simulink model "motorcontrol_19a"  (R2019a)
settings: Solver=FixedStepDiscrete  StartTime=0.0  StopTime=20  FixedStep=Ts.simulink  MaxStep=5e-5  RelTol=1e-3  EnableMultiTasking=on
undefined symbols (not defined in the file): ControllerMode, ControlMode, ctrlParams, dataType, DiscIntNeverNeededParam, inverter, NumBits1, NumBits2, PI_params, pmsm, Slope1, Slope2, Ts
libraries: simulink x17
(part 2 of 3)

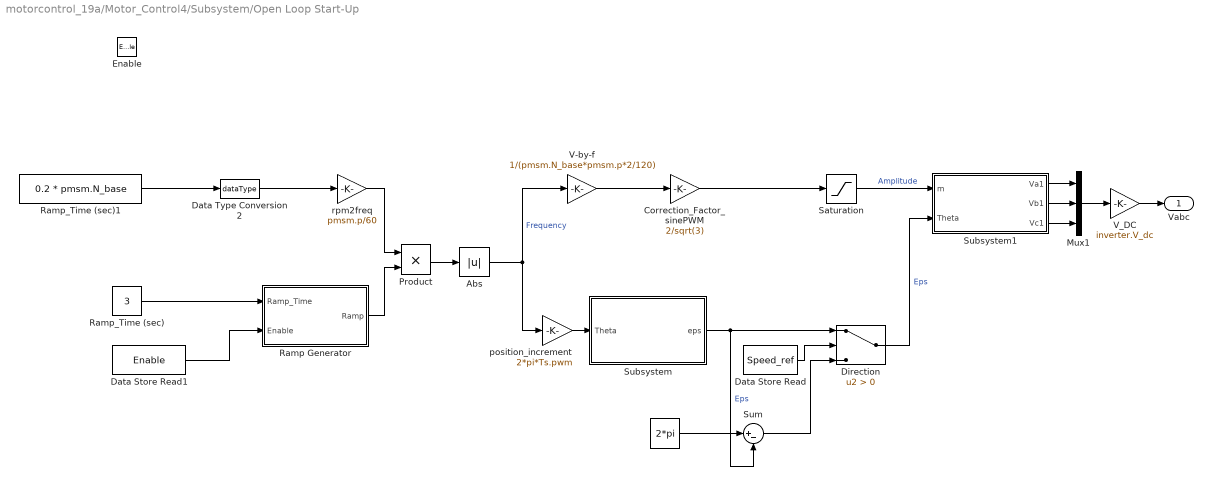
== system motorcontrol_19a/Motor_Control4/Subsystem/Open Loop Start-Up ==
  Enable : EnablePort  StatesWhenEnabling=reset
  " " : Constant  Value=2*pi  OutDataTypeStr=dataType  SampleTime=-1
  Abs : Abs
  Correction_Factor_sinePWM : Gain  Gain=2/sqrt(3)  RndMeth=Simplest  OutDataTypeStr=Inherit: Same as input
  Data Store Read : DataStoreRead  DataStoreName=Speed_ref
  Data Store Read1 : DataStoreRead  DataStoreName=Enable
  Data Type Conversion2 : DataTypeConversion  OutDataTypeStr=dataType  RndMeth=Simplest
  Direction : Switch  Criteria=u2 > Threshold  OutDataTypeStr=dataType  RndMeth=Simplest
  Mux1 : Mux  Inputs=3
  Product : Product  RndMeth=Simplest  OutDataTypeStr=Inherit: Same as first input
  Ramp Generator : Subsystem
  Ramp_Time (sec) : Constant  Value=3  OutDataTypeStr=dataType  SampleTime=-1
  Ramp_Time (sec)1 : Constant  Value=0.2 * pmsm.N_base  OutDataTypeStr=dataType  SampleTime=-1
  Saturation : Saturate  UpperLimit=0.95  LowerLimit=0.15  RndMeth=Simplest
  Subsystem : Subsystem  mask(Position Generator){Offset=0, InitialCondition=0}
      mask prompts: Offset "Initial Theta output:"; InitialCondition "Initial condition"
      mask help:
      | <p>Generate position ramp of required frequency.
      | <br><br>
      | The block accepts position increment and outputs position ramp.
      | <br>
      | The position increment for required frequency (Hz) can be computed by following:
      | <br><br>
      | &Delta;&theta; (per-unit) = Frequency&#8231;Sample Time
      | <br>
      | &Delta;&theta; (radians)&nbsp; = 2&#8231;&pi;&#8231;Frequency&#8231;Sample Time
      | <br>
      | &Delta;&theta; (degrees) = 360&#8231;Frequency&#8231;Sample Time <br>
      mask Display: fprintf('Position\n Generator');
  Subsystem1 : Subsystem  mask(3-Phase Sine Voltage Generator){}
      mask help:
      | Generate balanced 3-phase sinusoidal signals described by magnitude and position inputs.
      |
      | The block accepts voltage reference by magnitude and position inputs, and outputs balanced three phase sinusoidal voltages of frequency corresponding to position input.
      |
      | Enter position input units and number of data points for sine-cosine look-up table.
      mask Display: fprintf('3-Phase Sine\n  Voltage Generator');
  Sum : Sum  Inputs=|+-  RndMeth=Simplest  OutDataTypeStr=Inherit: Same as first input
  V-by-f : Gain  Gain=1/(pmsm.N_base*pmsm.p*2/120)  RndMeth=Simplest  OutDataTypeStr=Inherit: Same as input
  V_DC : Gain  Gain=inverter.V_dc
  position_increment : Gain  Gain=2*pi*Ts.pwm  RndMeth=Simplest  OutDataTypeStr=Inherit: Same as input
  rpm2freq : Gain  Gain=pmsm.p/60  RndMeth=Simplest  OutDataTypeStr=Inherit: Same as input
  Vabc : Outport  VectorParamsAs1DForOutWhenUnconnected=off
  wires:
  V_DC/1 -> Vabc/1
  Data Store Read/1 -> Direction/2
  Ramp_Time (sec)1/1 -> Data Type Conversion2/1
  Data Type Conversion2/1 -> rpm2freq/1
  Correction_Factor_sinePWM/1 -> Saturation/1
  Data Store Read1/1 -> Ramp Generator/2(Enable)
  rpm2freq/1 -> Product/1
  Product/1 -> Abs/1
  V-by-f/1 -> Correction_Factor_sinePWM/1
  position_increment/1 -> Subsystem/1(Theta)
  Abs/1 -> V-by-f/1, position_increment/1  "Frequency"
  Sum/1 -> Direction/3
  " "/1 -> Sum/1
  Subsystem/1(eps) -> Direction/1, Sum/2  "Eps"
  Ramp_Time (sec)/1 -> Ramp Generator/1(Ramp_Time)
  Ramp Generator/1(Ramp) -> Product/2
  Mux1/1 -> V_DC/1
  Saturation/1 -> Subsystem1/1(m)  "Amplitude"
  Direction/1 -> Subsystem1/2(Theta)  "Eps"
  Subsystem1/2(Vb1) -> Mux1/2
  Subsystem1/1(Va1) -> Mux1/1
  Subsystem1/3(Vc1) -> Mux1/3

== system motorcontrol_19a/Subsystem/Simulation/Data_Type_Float ==
  In1 : Inport
  In2 : Inport  Port=2
  Data Type Conversion2 : DataTypeConversion  OutDataTypeStr=dataType  RndMeth=Simplest
  Mux : Mux  Inputs=2
  Data : Outport
  wires:
  Data Type Conversion2/1 -> Mux/2
  In2/1 -> Data Type Conversion2/1
  Mux/1 -> Data/1
  In1/1 -> Mux/1

== system motorcontrol_19a/Subsystem/Simulation/Parse ==
  Enable_PWM : Inport
  Bitwise Operator : simulink/Logic and Bit Operations/Bitwise Operator  logicop=AND  UseBitMask=on  BitMask=hex2dec('0001')  BitMaskRealWorld=Stored Integer
  Data : Outport
  wires:
  Enable_PWM/1 -> Bitwise Operator/1
  Bitwise Operator/1 -> Data/1

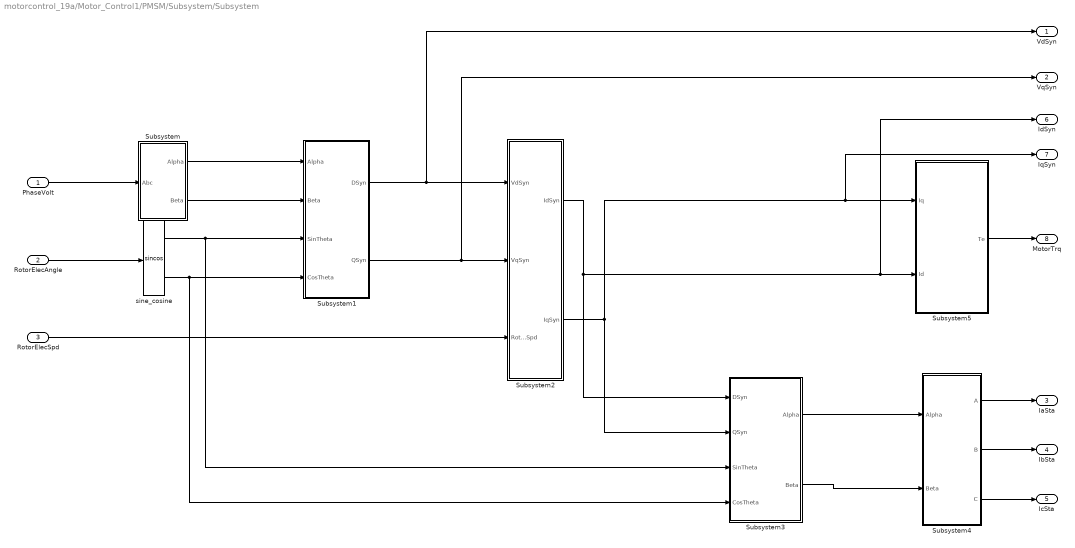
== system motorcontrol_19a/Motor_Control1/PMSM/Subsystem/Subsystem ==
  PhaseVolt : Inport
  RotorElecAngle : Inport  Port=2
  RotorElecSpd : Inport  Port=3
  Subsystem : Subsystem
  Subsystem1 : Subsystem
  Subsystem2 : Subsystem
  Subsystem3 : Subsystem
  Subsystem4 : Subsystem
  Subsystem5 : Subsystem
  sine_cosine : Trigonometry  Operator=sincos
  VdSyn : Outport  VectorParamsAs1DForOutWhenUnconnected=off
  VqSyn : Outport  Port=2  VectorParamsAs1DForOutWhenUnconnected=off
  IaSta : Outport  Port=3  VectorParamsAs1DForOutWhenUnconnected=off
  IbSta : Outport  Port=4  VectorParamsAs1DForOutWhenUnconnected=off
  IcSta : Outport  Port=5  VectorParamsAs1DForOutWhenUnconnected=off
  IdSyn : Outport  Port=6  VectorParamsAs1DForOutWhenUnconnected=off
  IqSyn : Outport  Port=7  VectorParamsAs1DForOutWhenUnconnected=off
  MotorTrq : Outport  Port=8  VectorParamsAs1DForOutWhenUnconnected=off
  wires:
  Subsystem4/2(B) -> IbSta/1
  Subsystem5/1(Te) -> MotorTrq/1
  Subsystem3/1(Alpha) -> Subsystem4/1(Alpha)
  Subsystem4/3(C) -> IcSta/1
  sine_cosine/1 -> Subsystem3/3(SinTheta), Subsystem1/3(SinTheta)
  Subsystem1/2(QSyn) -> VqSyn/1, Subsystem2/2(VqSyn)
  Subsystem3/2(Beta) -> Subsystem4/2(Beta)
  Subsystem2/2(IqSyn) -> IqSyn/1, Subsystem5/1(Iq), Subsystem3/2(QSyn)
  Subsystem4/1(A) -> IaSta/1
  RotorElecSpd/1 -> Subsystem2/3(RotorElecSpd)
  Subsystem/1(Alpha) -> Subsystem1/1(Alpha)
  Subsystem1/1(DSyn) -> Subsystem2/1(VdSyn), VdSyn/1
  Subsystem/2(Beta) -> Subsystem1/2(Beta)
  RotorElecAngle/1 -> sine_cosine/1
  sine_cosine/2 -> Subsystem3/4(CosTheta), Subsystem1/4(CosTheta)
  PhaseVolt/1 -> Subsystem/1(Abc)
  Subsystem2/1(IdSyn) -> Subsystem3/1(DSyn), IdSyn/1, Subsystem5/2(Id)

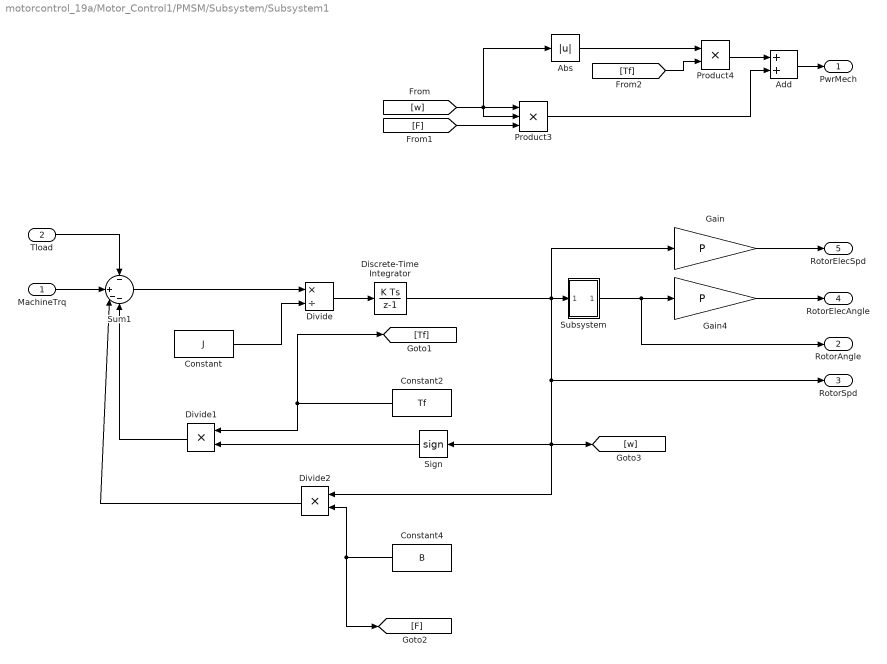
== system motorcontrol_19a/Motor_Control1/PMSM/Subsystem/Subsystem1 ==
  MachineTrq : Inport
  Tload : Inport  Port=2
  Abs : Abs
  Add : Sum
  Constant : Constant  Value=J  OutDataTypeStr=Inherit: Inherit via back propagation  SampleTime=-1
  Constant2 : Constant  Value=Tf  OutDataTypeStr=Inherit: Inherit via back propagation  SampleTime=-1
  Constant4 : Constant  Value=B  OutDataTypeStr=Inherit: Inherit via back propagation  SampleTime=-1
  Discrete-Time Integrator : DiscreteIntegrator  InitialCondition=omega_init  SampleTime=Ts  OutDataTypeStr=single  LimitOutput=on  UpperSaturationLimit=10e6  LowerSaturationLimit=-10e6  ICPrevOutput=DiscIntNeverNeededParam  ICPrevScaledInput=DiscIntNeverNeededParam
  Divide : Product  Inputs=*/  OutDataTypeStr=Inherit: Same as first input
  Divide1 : Product  Inputs=**
  Divide2 : Product  Inputs=**
  Gain : Gain  Gain=P  SaturateOnIntegerOverflow=on  OutDataTypeStr=Inherit: Same as input  ParamDataTypeStr=Inherit: Same as input
  Gain4 : Gain  Gain=P  SaturateOnIntegerOverflow=on  OutDataTypeStr=Inherit: Same as input  ParamDataTypeStr=Inherit: Same as input
  Product3 : Product  Inputs=3  OutDataTypeStr=Inherit: Inherit via back propagation
  Product4 : Product
  Sign : Signum
  Subsystem : Subsystem  mask{Ts=Ts, Ic=theta_init, U=pi, L=-pi}
      mask prompts: Ts "Sample Time:"; Ic "Initial Condition:"; U "Upper Limit:"; L "Lower Limit:"
  Sum1 : Sum  Inputs=-|+--
  PwrMech : Outport  VectorParamsAs1DForOutWhenUnconnected=off
  RotorAngle : Outport  Port=2  VectorParamsAs1DForOutWhenUnconnected=off
  RotorSpd : Outport  Port=3  VectorParamsAs1DForOutWhenUnconnected=off
  RotorElecAngle : Outport  Port=4  VectorParamsAs1DForOutWhenUnconnected=off
  RotorElecSpd : Outport  Port=5  VectorParamsAs1DForOutWhenUnconnected=off
  wires:
  Divide1/1 -> Sum1/4
  Subsystem/1(Out1) -> RotorAngle/1, Gain4/1
  MachineTrq/1 -> Sum1/2
  [w] -> Product3/1, Product3/2, Abs/1
  Divide/1 -> Discrete-Time Integrator/1
  Tload/1 -> Sum1/1
  Add/1 -> PwrMech/1
  Divide2/1 -> Sum1/3
  Sign/1 -> Divide1/2
  Product3/1 -> Add/2
  Gain4/1 -> RotorElecAngle/1
  Sum1/1 -> Divide/1
  [Tf] -> Product4/2
  Discrete-Time Integrator/1 -> Subsystem/1(In1), RotorSpd/1, Sign/1, Divide2/1, [w], Gain/1
  Gain/1 -> RotorElecSpd/1
  Constant2/1 -> [Tf], Divide1/1
  Constant4/1 -> Divide2/2, [F]
  Abs/1 -> Product4/1
  Product4/1 -> Add/1
  [F] -> Product3/3
  Constant/1 -> Divide/2

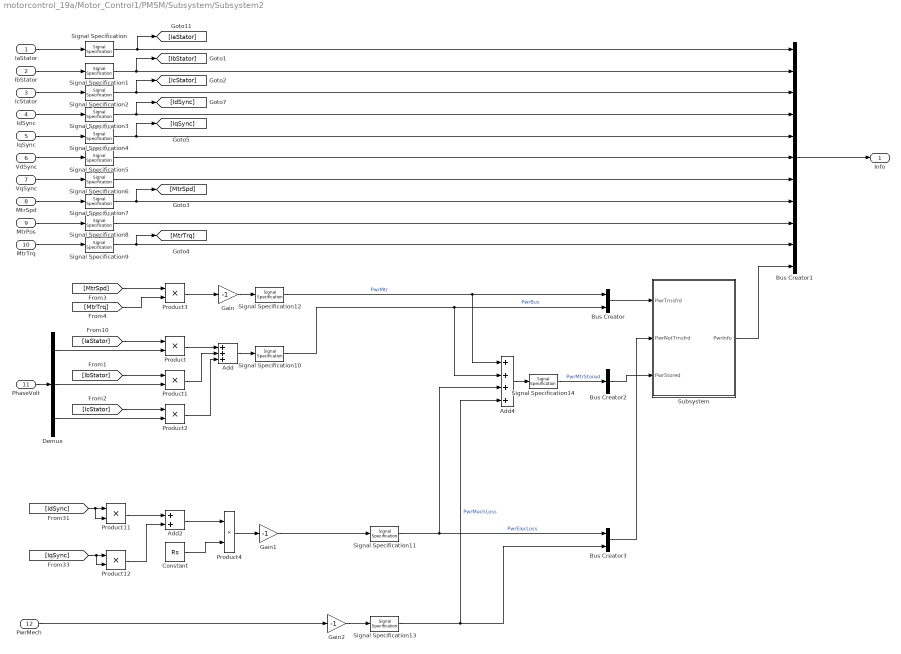
== system motorcontrol_19a/Motor_Control1/PMSM/Subsystem/Subsystem2 ==
  IaStator : Inport
  IbStator : Inport  Port=2
  IcStator : Inport  Port=3
  IdSync : Inport  Port=4
  IqSync : Inport  Port=5
  VdSync : Inport  Port=6
  VqSync : Inport  Port=7
  MtrSpd : Inport  Port=8
  MtrPos : Inport  Port=9
  MtrTrq : Inport  Port=10
  PhaseVolt : Inport  Port=11
  PwrMech : Inport  Port=12
  Add : Sum  Inputs=+++
  Add2 : Sum
  Add4 : Sum  Inputs=++++
  Bus Creator : BusCreator  Inputs=2
  Bus Creator1 : BusCreator  Inputs=11
  Bus Creator2 : BusCreator  Inputs=1
  Bus Creator3 : BusCreator  Inputs=2
  Constant : Constant  Value=Rs  OutDataTypeStr=Inherit: Inherit via back propagation
  Demux : Demux  Outputs=3
  Gain : Gain  Gain=-1  OutDataTypeStr=Inherit: Same as input
  Gain1 : Gain  Gain=-1  OutDataTypeStr=Inherit: Same as input
  Gain2 : Gain  Gain=-1  OutDataTypeStr=Inherit: Same as input
  Product{,1..3,11..12} (6 alike) : Product
  Product4 : Product  OutDataTypeStr=Inherit: Same as first input
  Signal Specification{,1..4} (5 alike) : SignalSpecification  Unit=A
  Signal Specification{10..14} (5 alike) : SignalSpecification  Unit=W
  Signal Specification5 : SignalSpecification  Unit=V
  Signal Specification6 : SignalSpecification  Unit=V
  Signal Specification7 : SignalSpecification  Unit=rad/s
  Signal Specification8 : SignalSpecification  Unit=rad
  Signal Specification9 : SignalSpecification  Unit=N*m
  Subsystem : Subsystem
  Info : Outport  VectorParamsAs1DForOutWhenUnconnected=off
  wires:
  Signal Specification2/1 -> Bus Creator1/3, [IcStator]
  [MtrSpd] -> Product3/1
  MtrPos/1 -> Signal Specification8/1
  Gain/1 -> Signal Specification12/1
  Signal Specification4/1 -> Bus Creator1/5, [IqSync]
  [IdSync] -> Product11/1, Product11/2
  Signal Specification11/1 -> Bus Creator3/1, Add4/3  "PwrElecLoss"
  Signal Specification14/1 -> Bus Creator2/1  "PwrMtrStored"
  [IqSync] -> Product12/1, Product12/2
  MtrSpd/1 -> Signal Specification7/1
  MtrTrq/1 -> Signal Specification9/1
  VqSync/1 -> Signal Specification6/1
  IaStator/1 -> Signal Specification/1
  Demux/3 -> Product2/2
  [IcStator] -> Product2/1
  Signal Specification12/1 -> Bus Creator/1, Add4/1  "PwrMtr"
  IcStator/1 -> Signal Specification2/1
  Signal Specification5/1 -> Bus Creator1/6
  IqSync/1 -> Signal Specification4/1
  IdSync/1 -> Signal Specification3/1
  Bus Creator1/1 -> Info/1
  Signal Specification9/1 -> Bus Creator1/10, [MtrTrq]
  Signal Specification3/1 -> Bus Creator1/4, [IdSync]
  Signal Specification6/1 -> Bus Creator1/7
  PhaseVolt/1 -> Demux/1
  Signal Specification8/1 -> Bus Creator1/9
  Product2/1 -> Add/3
  [IaStator] -> Product/1
  Add2/1 -> Product4/1
  [IbStator] -> Product1/1
  Bus Creator3/1 -> Subsystem/2(PwrNotTrnsfrd)
  Add/1 -> Signal Specification10/1
  Demux/2 -> Product1/2
  Product1/1 -> Add/2
  Product/1 -> Add/1
  Signal Specification/1 -> Bus Creator1/1, [IaStator]
  Signal Specification7/1 -> Bus Creator1/8, [MtrSpd]
  Signal Specification1/1 -> Bus Creator1/2, [IbStator]
  Subsystem/1(PwrInfo) -> Bus Creator1/11
  VdSync/1 -> Signal Specification5/1
  [MtrTrq] -> Product3/2
  Gain1/1 -> Signal Specification11/1
  IbStator/1 -> Signal Specification1/1
  Bus Creator/1 -> Subsystem/1(PwrTrnsfrd)
  Product3/1 -> Gain/1
  Signal Specification10/1 -> Bus Creator/2, Add4/2  "PwrBus"
  Gain2/1 -> Signal Specification13/1
  Add4/1 -> Signal Specification14/1
  PwrMech/1 -> Gain2/1
  Signal Specification13/1 -> Bus Creator3/2, Add4/4  "PwrMechLoss"
  Product11/1 -> Add2/1
  Constant/1 -> Product4/2
  Product12/1 -> Add2/2
  Product4/1 -> Gain1/1
  Demux/1 -> Product/2
  Bus Creator2/1 -> Subsystem/3(PwrStored)

== system motorcontrol_19a/Motor_Control4/Input Scaling/ Calculate Position and Speed/IndexFinder ==
  In1 : Inport
  Enable : EnablePort
  AND : Logic  AllPortsSameDT=off  OutDataTypeStr=boolean
  Compare To Constant : simulink/Logic and Bit Operations/Compare To Constant  relop===  const=0  OutDataTypeStr=boolean
  Compare To Constant1 : simulink/Logic and Bit Operations/Compare To Constant  relop=>  const=0  OutDataTypeStr=boolean
  Delay3 : Delay  DelayLength=1
  Out1 : Outport
  wires:
  AND/1 -> Out1/1
  Delay3/1 -> Compare To Constant/1
  Compare To Constant/1 -> AND/1
  Compare To Constant1/1 -> AND/2
  In1/1 -> Compare To Constant1/1, Delay3/1

== system motorcontrol_19a/Motor_Control4/Input Scaling/ Calculate Position and Speed/Subsystem ==
  x : Inport
  Add : Sum
  Add1 : Sum  Inputs=-+
  Constant : Constant  OutDataTypeStr=single  SampleTime=-1
  Data Type Duplicate : DataTypeDuplicate  NumInputPorts=3
  Filter_Constant : Constant  Value=FilterConstant  OutDataTypeStr=single  SampleTime=-1
  Product : Product  RndMeth=Simplest  OutDataTypeStr=Inherit: Same as first input
  Product1 : Product  RndMeth=Simplest  OutDataTypeStr=Inherit: Same as first input
  Unit Delay : UnitDelay  SampleTime=-1  HasFrameUpgradeWarning=on
  y : Outport
  wires:
  x/1 -> Product/1, Data Type Duplicate/1
  Filter_Constant/1 -> Product/2, Add1/1, Data Type Duplicate/2
  Product/1 -> Add/1
  Add/1 -> y/1, Unit Delay/1
  Product1/1 -> Add/2
  Unit Delay/1 -> Product1/2
  Add1/1 -> Product1/1
  Constant/1 -> Data Type Duplicate/3, Add1/2

== system motorcontrol_19a/Motor_Control4/Input Scaling/ Calculate Position and Speed/Subsystem1 ==
  note: Speed measurement
  Position : Inport
  Delay : Delay  DelayLength=DelayLength  UseCircularBuffer=on
  SpeedCount : Sum  Inputs=+-|  OutDataTypeStr=int32  RndMeth=Simplest
  SpeedGain : Gain  Gain=single(2*pi)/(DelayLength*SampleTimeAsync(1)*4294967296)  ParamDataTypeStr=single  OutDataTypeStr=single  RndMeth=Simplest
  SpeedToCount : Gain  Gain=uint32(4294967296/6.2832)  ParamDataTypeStr=uint32  OutDataTypeStr=uint32  RndMeth=Simplest
  Speed : Outport  VectorParamsAs1DForOutWhenUnconnected=off
  wires:
  Position/1 -> SpeedToCount/1
  Delay/1 -> SpeedCount/2
  SpeedGain/1 -> Speed/1
  SpeedToCount/1 -> Delay/1, SpeedCount/1
  SpeedCount/1 -> SpeedGain/1

== system motorcontrol_19a/Motor_Control4/Input Scaling/ Calculate Position and Speed/Subsystem2 ==
  note: PositionComputation
  Count : Inport  OutDataTypeStr=uint16
  IndexCount : Inport  Port=2  OutDataTypeStr=uint16
  If1 : If
  Merge : Merge
  PositionGain : Gain  Gain=single(2*pi)/single(EncoderSlitsPerRevolution*4)  ParamDataTypeStr=single  OutDataTypeStr=single  RndMeth=Simplest
  PositionNoReset : Subsystem  TreatAsAtomicUnit=on
  PositionResetatIndex : Subsystem  TreatAsAtomicUnit=on
  ResetMode : Constant  OutDataTypeStr=int16
  Position : Outport  VectorParamsAs1DForOutWhenUnconnected=off
  wires:
  If1/2 -> PositionResetatIndex/Action
  If1/1 -> PositionNoReset/Action
  PositionGain/1 -> Position/1
  Merge/1 -> PositionGain/1
  ResetMode/1 -> If1/1
  PositionResetatIndex/1(Position) -> Merge/2
  Count/1 -> PositionNoReset/2(Count), PositionResetatIndex/1(Count)
  PositionNoReset/1(Position) -> Merge/1
  IndexCount/1 -> PositionNoReset/1(Index)

== system motorcontrol_19a/Motor_Control4/Input Scaling/ Calculate Position and Speed/Subsystem3 ==
  ϴm : Inport  OutMin=0  OutMax=maxAngleIn
  Offset : Inport  Port=2  OutMin=0  OutMax=1
  Data Type Duplicate : DataTypeDuplicate
  Subsystem : Subsystem
  Subsystem1 : Subsystem
  ϴe : Outport  VectorParamsAs1DForOutWhenUnconnected=off
  wires:
  Offset/1 -> Subsystem/2(In2)
  Subsystem1/2(ϴe) -> ϴe/1
  Subsystem1/1(Out1) -> Data Type Duplicate/2
  ϴm/1 -> Data Type Duplicate/1, Subsystem/1(ϴm)
  Subsystem/1(Out1) -> Subsystem1/1(In1)

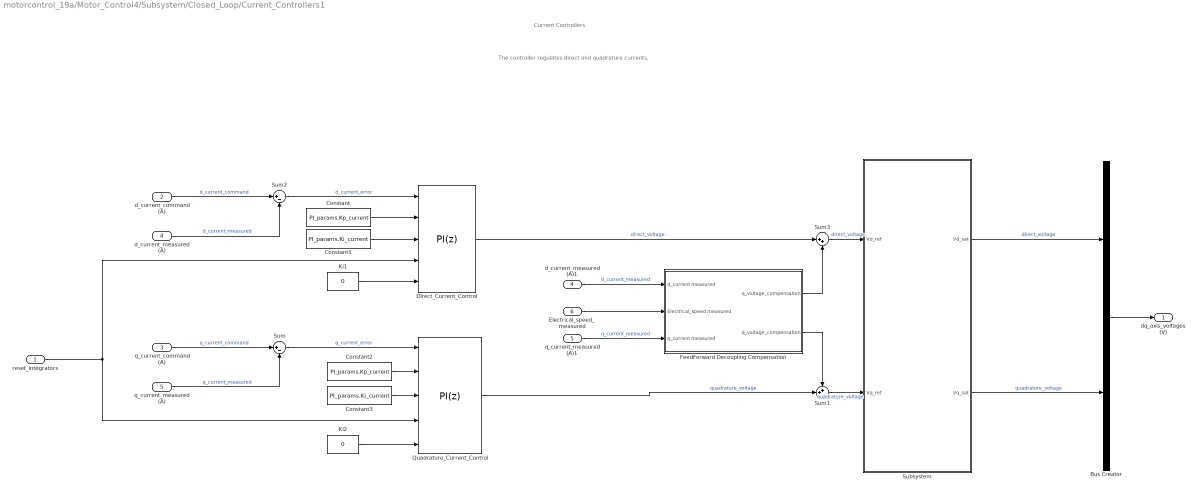
== system motorcontrol_19a/Motor_Control4/Subsystem/Closed_Loop/Current_Controllers1 ==
  note: Current Controllers
  note: The controller regulates direct and quadrature currents.
  reset_integrators : Inport
  d_current_command (A) : Inport  Port=2
  q_current_command (A) : Inport  Port=3
  d_current_measured (A) : Inport  Port=4
  q_current_measured (A) : Inport  Port=5
  Electrical_speed_measured : Inport  Port=6
  Bus Creator : BusCreator  Inputs=2
  Constant : Constant  Value=PI_params.Kp_current  OutDataTypeStr=dataType  SampleTime=-1
  Constant1 : Constant  Value=PI_params.Ki_current  OutDataTypeStr=dataType  SampleTime=-1
  Constant2 : Constant  Value=PI_params.Kp_current  OutDataTypeStr=dataType  SampleTime=-1
  Constant3 : Constant  Value=PI_params.Ki_current  OutDataTypeStr=dataType  SampleTime=-1
  Direct_Current_Control : simulink/Continuous/PID Controller  Controller=PI  Form=Parallel  TimeDomain=Discrete-time  SampleTime=-1  IntegratorMethod=Forward Euler  FilterMethod=Forward Euler  ControllerParametersSource=external  P=ctrlParams.Current_P  I=ctrlParams.Current_I  D=0  UseFilter=on  N=100  TunerSelectOption=Transfer Function Based (PID Tuner App)  InitialConditionSource=external  InitialConditionForIntegrator=0  InitialConditionForFilter=0  DifferentiatorICPrevScaledInput=0  ExternalReset=level  TrackingMode=off  Kt=1  LimitOutput=on  UpperSaturationLimit=inverter.V_dc  LowerSaturationLimit=-inverter.V_dc  LinearizeAsGain=off  AntiWindupMode=clamping  Kb=0  POutMin=[]  POutMax=[]  IOutMin=[]  IOutMax=[]  DOutMin=[]  DOutMax=[]  NOutMin=[]  NOutMax=[]  SumOutMin=[]  SumOutMax=[]  SaturationOutMin=[]  SaturationOutMax=[]  PParamMin=[]  PParamMax=[]  IParamMin=[]  IParamMax=[]  DParamMin=[]  DParamMax=[]  NParamMin=[]  NParamMax=[]  KbParamMin=[]  KbParamMax=[]  KtParamMin=[]  KtParamMax=[]  KbOutMin=[]  KbOutMax=[]  KtOutMin=[]  KtOutMax=[]  IntegratorOutMin=[]  IntegratorOutMax=[]  FilterOutMin=[]  FilterOutMax=[]  SumI1OutMin=[]  SumI1OutMax=[]  SumI2OutMin=[]  SumI2OutMax=[]  SumI3OutMin=[]  SumI3OutMax=[]  SumI4OutMin=[]  SumI4OutMax=[]  SumDOutMin=[]  SumDOutMax=[]  DifferentiatorOutMin=[]  DifferentiatorOutMax=[]  FilterDiffOutCoefMin=[]  FilterDiffOutCoefMax=[]  ReciprocalOutMin=[]  ReciprocalOutMax=[]  SumDenOutMin=[]  SumDenOutMax=[]  SumNumOutMin=[]  SumNumOutMax=[]  DivideOutMin=[]  DivideOutMax=[]  IntegratorContinuousStateAttributes=''  IntegratorStateMustResolveToSignalObject=off  IntegratorRTWStateStorageClass=Auto  FilterContinuousStateAttributes=''  FilterStateMustResolveToSignalObject=off  FilterRTWStateStorageClass=Auto  ParallelPVariant=ExternalParameters  IdealPVariant=Disabled  IVariant=ExternalParameters  DVariant=Disabled  IntegratorVariant=Discrete  SatVariant=Enabled  AWVariant=DiscClampingParallel  PCopyVariant=Disabled  TRVariant=Disabled  FdbkBlocksVariant=Forward  IdealPFdbkVariant=Disabled  SatFdbkVariant=Disabled  DerivativeFilterVariant=Disabled  NVariant=Disabled  NCopyVariant=Disabled_SignalSpec  FilterICVariant=Disabled  IntegratorICVariant=ExternalICs  ExternalResetVariant=ExternalReset  TRSumVariant=Passthrough  SumFdbkVariant=Disabled  SumVariant=Sum_PI
      settings: AttributesFormatString=%<AntiWindupMode>
  FeedForward Decoupling Compensation : Subsystem
      mask Display: fprintf('Feed-forward \n Decoupling')
  Ki1 : Constant  Value=0  OutDataTypeStr=dataType  SampleTime=-1
  Ki2 : Constant  Value=0  OutDataTypeStr=dataType  SampleTime=-1
  Quadrature_Current_Control : simulink/Continuous/PID Controller  Controller=PI  Form=Parallel  TimeDomain=Discrete-time  SampleTime=-1  IntegratorMethod=Forward Euler  FilterMethod=Forward Euler  ControllerParametersSource=external  P=ctrlParams.Current_P  I=ctrlParams.Current_I  D=0  UseFilter=on  N=100  TunerSelectOption=Transfer Function Based (PID Tuner App)  InitialConditionSource=external  InitialConditionForIntegrator=0  InitialConditionForFilter=0  DifferentiatorICPrevScaledInput=0  ExternalReset=level  TrackingMode=off  Kt=1  LimitOutput=on  UpperSaturationLimit=inverter.V_dc  LowerSaturationLimit=-inverter.V_dc  LinearizeAsGain=off  AntiWindupMode=clamping  Kb=0  POutMin=[]  POutMax=[]  IOutMin=[]  IOutMax=[]  DOutMin=[]  DOutMax=[]  NOutMin=[]  NOutMax=[]  SumOutMin=[]  SumOutMax=[]  SaturationOutMin=[]  SaturationOutMax=[]  PParamMin=[]  PParamMax=[]  IParamMin=[]  IParamMax=[]  DParamMin=[]  DParamMax=[]  NParamMin=[]  NParamMax=[]  KbParamMin=[]  KbParamMax=[]  KtParamMin=[]  KtParamMax=[]  KbOutMin=[]  KbOutMax=[]  KtOutMin=[]  KtOutMax=[]  IntegratorOutMin=[]  IntegratorOutMax=[]  FilterOutMin=[]  FilterOutMax=[]  SumI1OutMin=[]  SumI1OutMax=[]  SumI2OutMin=[]  SumI2OutMax=[]  SumI3OutMin=[]  SumI3OutMax=[]  SumI4OutMin=[]  SumI4OutMax=[]  SumDOutMin=[]  SumDOutMax=[]  DifferentiatorOutMin=[]  DifferentiatorOutMax=[]  FilterDiffOutCoefMin=[]  FilterDiffOutCoefMax=[]  ReciprocalOutMin=[]  ReciprocalOutMax=[]  SumDenOutMin=[]  SumDenOutMax=[]  SumNumOutMin=[]  SumNumOutMax=[]  DivideOutMin=[]  DivideOutMax=[]  IntegratorContinuousStateAttributes=''  IntegratorStateMustResolveToSignalObject=off  IntegratorRTWStateStorageClass=Auto  FilterContinuousStateAttributes=''  FilterStateMustResolveToSignalObject=off  FilterRTWStateStorageClass=Auto  ParallelPVariant=ExternalParameters  IdealPVariant=Disabled  IVariant=ExternalParameters  DVariant=Disabled  IntegratorVariant=Discrete  SatVariant=Enabled  AWVariant=DiscClampingParallel  PCopyVariant=Disabled  TRVariant=Disabled  FdbkBlocksVariant=Forward  IdealPFdbkVariant=Disabled  SatFdbkVariant=Disabled  DerivativeFilterVariant=Disabled  NVariant=Disabled  NCopyVariant=Disabled_SignalSpec  FilterICVariant=Disabled  IntegratorICVariant=ExternalICs  ExternalResetVariant=ExternalReset  TRSumVariant=Passthrough  SumFdbkVariant=Disabled  SumVariant=Sum_PI
      settings: AttributesFormatString=%<AntiWindupMode>
  Subsystem : Subsystem  mask(DQ Limiter){Vmax=inverter.V_dc / sqrt(3)}
      mask prompts: Vmax "D-Q saturation limit:"
      mask help:
      | Implement saturation on reference dq voltages, with respect to phase voltage peak limit.
      |
      | The block accepts reference values of d and q axis voltages, and outputs corresponding saturated values along with unsaturated peak value to initiate field weakening control.
      |
      | Enter the phase voltage peak limit in the dialog box to initiate saturation.
      mask Display: fprintf('DQ Limiter');
  Sum : Sum  Inputs=|+-
  Sum1 : Sum  Inputs=++|
  Sum2 : Sum  Inputs=|+-
  Sum3 : Sum  Inputs=|++
  d_current_measured (A)1 : InportShadow  Port=4
  q_current_measured (A)1 : InportShadow  Port=5
  dq_axis_voltages (V) : Outport
  wires:
  d_current_command (A)/1 -> Sum2/1  "d_current_command"
  Bus Creator/1 -> dq_axis_voltages (V)/1
  q_current_command (A)/1 -> Sum/1  "q_current_command"
  Sum2/1 -> Direct_Current_Control/1  "d_current_error"
  Sum/1 -> Quadrature_Current_Control/1  "q_current_error"
  reset_integrators/1 -> Direct_Current_Control/4, Quadrature_Current_Control/4
  d_current_measured (A)/1 -> Sum2/2  "d_current_measured"
  q_current_measured (A)/1 -> Sum/2  "q_current_measured"
  Quadrature_Current_Control/1 -> Sum1/2  "quadrature_voltage"
  FeedForward Decoupling Compensation/2(d_voltage_compensation) -> Sum1/1
  Direct_Current_Control/1 -> Sum3/1  "direct_voltage"
  FeedForward Decoupling Compensation/1(q_voltage_compensation) -> Sum3/2
  d_current_measured (A)1/1 -> FeedForward Decoupling Compensation/1(d_current measured)  "d_current_measured"
  q_current_measured (A)1/1 -> FeedForward Decoupling Compensation/3(q_current measured)  "q_current_measured"
  Electrical_speed_measured/1 -> FeedForward Decoupling Compensation/2(Electrical_speed measured)
  Subsystem/2(Vq_sat) -> Bus Creator/2  "quadrature_voltage"
  Subsystem/1(Vd_sat) -> Bus Creator/1  "direct_voltage"
  Sum3/1 -> Subsystem/1(Vd_ref)  "direct_voltage"
  Sum1/1 -> Subsystem/2(Vq_ref)  "quadrature_voltage"
  Constant/1 -> Direct_Current_Control/2
  Constant1/1 -> Direct_Current_Control/3
  Constant2/1 -> Quadrature_Current_Control/2
  Constant3/1 -> Quadrature_Current_Control/3
  Ki1/1 -> Direct_Current_Control/5
  Ki2/1 -> Quadrature_Current_Control/5

== system motorcontrol_19a/Motor_Control4/Subsystem/Closed_Loop/Sine-Cosine Lookup ==
  Theta : Inport
  Data Type Duplicate : DataTypeDuplicate  NumInputPorts=4
  Data Type Propagation : simulink/Signal Attributes/Data Type Propagation  PropDataType=fixdt(1, 16)  IfRefDouble=double  IfRefSingle=single  IsSigned=IsSigned1 or IsSigned2  NumBitsBase=max([NumBits1 NumBits2])  NumBitsMult=1  NumBitsAdd=0  NumBitsAllowFinal=1:128  PropScalingMode=Obtain via best precision  PropScaling=2^-10  ValuesUsedBestPrec=[0 dlgSett.index_gain]  SlopeBase=min([Slope1 Slope2])  SlopeMult=1  SlopeAdd=0  BiasBase=Bias1  BiasMult=1  BiasAdd=0
      settings: SourceProductBaseCode=SL
  Data Type Conversion1 : DataTypeConversion  RndMeth=Simplest
  Get_FractionVal : DataTypeConversion  RndMeth=Simplest
  Get_Integer : DataTypeConversion  OutDataTypeStr=uint16  RndMeth=Simplest
  Lookup : Selector  IndexMode=Zero-based  InputPortWidth=dlgSett.size  IndexOptions=Index vector (port)  Indices=[1 3]  OutputSizes=1
  Subsystem : Subsystem
  Subsystem1 : Subsystem
  Sum : Sum  Inputs=|++  AccumDataTypeStr=uint32  OutDataTypeStr=uint32  RndMeth=Simplest
  Sum2 : Sum  Inputs=|+-  RndMeth=Simplest  OutDataTypeStr=Inherit: Same as first input
  indexing : Gain  Gain=dlgSett.index_gain  OutDataTypeStr=Inherit: Inherit via back propagation  RndMeth=Simplest
  offset : Constant  Value=[1 0 (dlgSett.Offset+1) dlgSett.Offset]  OutDataTypeStr=int16  SampleTime=-1
  sine_table_values : Constant  Value=dlgSett.sin_table  OutDataTypeStr=Inherit: Inherit via back propagation  SampleTime=-1
  sin : Outport  VectorParamsAs1DForOutWhenUnconnected=off
  cos : Outport  Port=2  VectorParamsAs1DForOutWhenUnconnected=off
  wires:
  Subsystem1/2(Out2) -> cos/1
  Data Type Conversion1/1 -> Sum2/2
  Subsystem1/1(Out1) -> sin/1
  offset/1 -> Sum/2
  Lookup/1 -> Subsystem1/1(In1), Data Type Duplicate/3
  Get_FractionVal/1 -> Subsystem1/2(In2), Data Type Duplicate/4
  Sum/1 -> Lookup/2
  Theta/1 -> Subsystem/1(In1), Data Type Propagation/1, Data Type Propagation/2, Data Type Duplicate/1
  indexing/1 -> Get_Integer/1, Data Type Propagation/3, Sum2/1
  sine_table_values/1 -> Data Type Duplicate/2, Lookup/1
  Get_Integer/1 -> Data Type Conversion1/1, Sum/1
  Sum2/1 -> Get_FractionVal/1
  Subsystem/1(Out1) -> indexing/1

== system motorcontrol_19a/Motor_Control4/Subsystem/Closed_Loop/Subsystem ==
  note: D-Current Command
  note: The controller regulates motor velocity using rotor velocity feedback compared to a commanded velocity.
      | The output of the controller is the quadrature-winding current command which is directly proportional to the electromagnetic torque of the motor.
      | Since the motor being controlled is a Permanent Magnet Synchronous Machine, the rotor flux linkage is fixed (determined by the magnets),
      | hence the commanded direct-winding current is always zero.
  Zero : Constant  Value=0  OutDataTypeStr=dataType  SampleTime=-1
  d_current_command : Outport  OutDataTypeStr=dataType
  wires:
  Zero/1 -> d_current_command/1

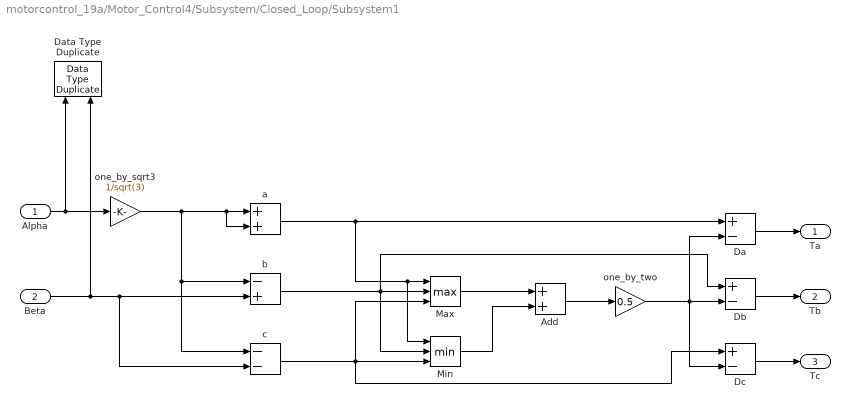
== system motorcontrol_19a/Motor_Control4/Subsystem/Closed_Loop/Subsystem1 ==
  Alpha : Inport
  Beta : Inport  Port=2
  Add : Sum  RndMeth=Simplest  OutDataTypeStr=Inherit: Same as first input
  Da : Sum  Inputs=+-  RndMeth=Simplest  OutDataTypeStr=Inherit: Same as first input
  Data Type Duplicate : DataTypeDuplicate
  Db : Sum  Inputs=+-  RndMeth=Simplest  OutDataTypeStr=Inherit: Same as first input
  Dc : Sum  Inputs=+-  RndMeth=Simplest  OutDataTypeStr=Inherit: Same as first input
  Max : MinMax  Function=max  Inputs=3  RndMeth=Simplest
  Min : MinMax  Inputs=3  RndMeth=Simplest
  a : Sum  RndMeth=Simplest  OutDataTypeStr=Inherit: Same as first input
  b : Sum  Inputs=-+  RndMeth=Simplest  OutDataTypeStr=Inherit: Same as first input
  c : Sum  Inputs=--  RndMeth=Simplest  OutDataTypeStr=Inherit: Same as first input
  one_by_sqrt3 : Gain  Gain=1/sqrt(3)  RndMeth=Simplest  OutDataTypeStr=Inherit: Same as input  ParamDataTypeStr=Inherit: Same as input
  one_by_two : Gain  Gain=0.5  RndMeth=Simplest  OutDataTypeStr=Inherit: Same as input  ParamDataTypeStr=Inherit: Same as input
  Ta : Outport  VectorParamsAs1DForOutWhenUnconnected=off
  Tb : Outport  Port=2  VectorParamsAs1DForOutWhenUnconnected=off
  Tc : Outport  Port=3  VectorParamsAs1DForOutWhenUnconnected=off
  wires:
  Da/1 -> Ta/1
  a/1 -> Da/1, Min/1, Max/1
  Max/1 -> Add/1
  Dc/1 -> Tc/1
  Min/1 -> Add/2
  one_by_two/1 -> Dc/2, Db/2, Da/2
  Alpha/1 -> one_by_sqrt3/1, Data Type Duplicate/1
  one_by_sqrt3/1 -> c/1, b/1, a/2, a/1
  Db/1 -> Tb/1
  Beta/1 -> Data Type Duplicate/2, b/2, c/2
  Add/1 -> one_by_two/1
  c/1 -> Max/3, Dc/1, Min/3
  b/1 -> Db/1, Min/2, Max/2

== system motorcontrol_19a/Motor_Control4/Subsystem/Closed_Loop/Subsystem2 ==
  a : Inport
  b : Inport  Port=2
  Data Type Duplicate : DataTypeDuplicate
  a_plus_2b : Sum  Inputs=+++  RndMeth=Simplest  OutDataTypeStr=Inherit: Same as first input
  one_by_sqrt3 : Gain  Gain=1/sqrt(3)  RndMeth=Simplest  OutDataTypeStr=Inherit: Same as input
  Alpha : Outport  VectorParamsAs1DForOutWhenUnconnected=off
  Beta : Outport  Port=2  VectorParamsAs1DForOutWhenUnconnected=off
  wires:
  a/1 -> a_plus_2b/1, Alpha/1, Data Type Duplicate/1
  a_plus_2b/1 -> one_by_sqrt3/1
  one_by_sqrt3/1 -> Beta/1
  b/1 -> a_plus_2b/2, a_plus_2b/3, Data Type Duplicate/2

== system motorcontrol_19a/Motor_Control4/Subsystem/Closed_Loop/Subsystem3 ==
  Alpha : Inport
  Beta : Inport  Port=2
  sine : Inport  Port=3
  cos : Inport  Port=4
  Data Type Duplicate : DataTypeDuplicate  NumInputPorts=4
  Subsystem : Subsystem
  acos : Product  RndMeth=Simplest  OutDataTypeStr=Inherit: Same as first input
  asin : Product  RndMeth=Simplest  OutDataTypeStr=Inherit: Same as first input
  bcos : Product  OutDataTypeStr=Inherit: Inherit via back propagation  RndMeth=Simplest
  bsin : Product  OutDataTypeStr=Inherit: Inherit via back propagation  RndMeth=Simplest
  sum_Ds : Sum  Inputs=|++  RndMeth=Simplest  OutDataTypeStr=Inherit: Same as first input
  sum_Qs : Sum  Inputs=|+-  RndMeth=Simplest  OutDataTypeStr=Inherit: Same as first input
  Ds : Outport  VectorParamsAs1DForOutWhenUnconnected=off
  Qs : Outport  Port=2  VectorParamsAs1DForOutWhenUnconnected=off
  wires:
  Alpha/1 -> Data Type Duplicate/1, acos/1, asin/1
  acos/1 -> sum_Ds/1
  sine/1 -> bsin/2, asin/2, Data Type Duplicate/4
  asin/1 -> sum_Qs/2
  Subsystem/2(q_axis) -> Qs/1
  Beta/1 -> Data Type Duplicate/2, bcos/1, bsin/1
  sum_Qs/1 -> Subsystem/2(q)
  bsin/1 -> sum_Ds/2
  cos/1 -> Data Type Duplicate/3, bcos/2, acos/2
  bcos/1 -> sum_Qs/1
  Subsystem/1(d_axis) -> Ds/1
  sum_Ds/1 -> Subsystem/1(d)

== system motorcontrol_19a/Motor_Control4/Subsystem/Closed_Loop/Subsystem4 ==
  Ds : Inport
  Qs : Inport  Port=2
  sin : Inport  Port=3
  cos : Inport  Port=4
  Data Type Duplicate : DataTypeDuplicate  NumInputPorts=4
  Subsystem : Subsystem
  dcos : Product  RndMeth=Simplest  OutDataTypeStr=Inherit: Same as first input
  dsin : Product  RndMeth=Simplest  OutDataTypeStr=Inherit: Same as first input
  qcos : Product  RndMeth=Simplest  OutDataTypeStr=Inherit: Same as first input
  qsin : Product  RndMeth=Simplest  OutDataTypeStr=Inherit: Same as first input
  sum_alpha : Sum  Inputs=|+-  RndMeth=Simplest  OutDataTypeStr=Inherit: Same as first input
  sum_beta : Sum  Inputs=|++  RndMeth=Simplest  OutDataTypeStr=Inherit: Same as first input
  Alpha : Outport  VectorParamsAs1DForOutWhenUnconnected=off
  Beta : Outport  Port=2  VectorParamsAs1DForOutWhenUnconnected=off
  wires:
  dsin/1 -> sum_beta/2
  sum_alpha/1 -> Subsystem/1(A)
  sin/1 -> Data Type Duplicate/4, qsin/2, dsin/2
  Subsystem/2(Beta) -> Beta/1
  Ds/1 -> Data Type Duplicate/1, dsin/1, dcos/1
  dcos/1 -> sum_alpha/1
  qcos/1 -> sum_beta/1
  sum_beta/1 -> Subsystem/2(B)
  Qs/1 -> Data Type Duplicate/2, qcos/1, qsin/1
  Subsystem/1(Alpha) -> Alpha/1
  qsin/1 -> sum_alpha/2
  cos/1 -> Data Type Duplicate/3, dcos/2, qcos/2

== system motorcontrol_19a/Motor_Control4/Subsystem/Open Loop Start-Up/Ramp Generator ==
  Ramp_Time : Inport
  Enable : Inport  Port=2
  Divide : Product  Inputs=*/  RndMeth=Simplest  OutDataTypeStr=Inherit: Same as first input
  NOT : Logic  Operator=NOT  IconShape=distinctive  AllPortsSameDT=off  OutDataTypeStr=boolean
  One : Constant  OutDataTypeStr=dataType  SampleTime=-1
  Ramp Generator : DiscreteIntegrator  IntegratorMethod=Accumulation: Forward Euler  gainval=1  ExternalReset=sampled level  SampleTime=-1  OutDataTypeStr=dataType  RndMeth=Simplest  LimitOutput=on  UpperSaturationLimit=1  LowerSaturationLimit=0  ICPrevOutput=DiscIntNeverNeededParam  ICPrevScaledInput=DiscIntNeverNeededParam
  Sample_Time : Gain  Gain=Ts.pwm  RndMeth=Simplest  OutDataTypeStr=Inherit: Same as input
  Ramp : Outport
  wires:
  NOT/1 -> Ramp Generator/2
  Enable/1 -> NOT/1
  Ramp_Time/1 -> Divide/2
  One/1 -> Divide/1
  Sample_Time/1 -> Ramp Generator/1
  Ramp Generator/1 -> Ramp/1  "Eps"
  Divide/1 -> Sample_Time/1

== system motorcontrol_19a/Motor_Control4/Subsystem/Open Loop Start-Up/Subsystem ==
  Theta : Inport
  " " : Constant  OutDataTypeStr=Inherit: Inherit via back propagation  SampleTime=-1
  Abs : Abs
  Data Type Duplicate : DataTypeDuplicate  NumInputPorts=4
  Data Type Duplicate1 : DataTypeDuplicate  NumInputPorts=3
  Data Type Conversion : DataTypeConversion  OutDataTypeStr=boolean  RndMeth=Simplest
  Direction : Switch  Criteria=u2 > Threshold  OutDataTypeStr=Inherit: Inherit via back propagation  RndMeth=Simplest
  Discrete-Time Integrator : DiscreteIntegrator  IntegratorMethod=Accumulation: Forward Euler  ExternalReset=sampled level  InitialConditionSource=external  SampleTime=-1  OutDataTypeStr=Inherit: Inherit via back propagation  RndMeth=Simplest  LimitOutput=on  UpperSaturationLimit=1  LowerSaturationLimit=0  ICPrevOutput=DiscIntNeverNeededParam  ICPrevScaledInput=DiscIntNeverNeededParam
  Frequency1 : Constant  OutDataTypeStr=Inherit: Inherit via back propagation  SampleTime=-1
  Ground_Reset : Ground
  Reset_Logic : Subsystem
  Sum2 : Sum  Inputs=|-+  RndMeth=Simplest  OutDataTypeStr=Inherit: Same as first input
  Theta_IncrementSource : Subsystem
  scale : Gain  Gain=2*pi  RndMeth=Simplest  OutDataTypeStr=Inherit: Same as input
  eps : Outport  VectorParamsAs1DForOutWhenUnconnected=off
  wires:
  Reset_Logic/1(Reset) -> Discrete-Time Integrator/2
  Theta/1 -> Theta_IncrementSource/1(In1), Direction/2
  Frequency1/1 -> Reset_Logic/2(One), Data Type Duplicate/2
  Reset_Logic/2(Initial_Condition) -> Discrete-Time Integrator/3, Data Type Duplicate/4
  Theta_IncrementSource/1(Out1) -> Abs/1
  scale/1 -> eps/1
  Discrete-Time Integrator/1 -> Reset_Logic/3(theta_e), Data Type Duplicate/3, Data Type Duplicate1/1, Direction/1, Sum2/1  "theta_e"
  Sum2/1 -> Direction/3
  Abs/1 -> Reset_Logic/1(freq*Ts), Data Type Duplicate/1, Discrete-Time Integrator/1
  Ground_Reset/1 -> Data Type Conversion/1
  Direction/1 -> scale/1, Data Type Duplicate1/3  "Eps"
  " "/1 -> Data Type Duplicate1/2, Sum2/2
  Data Type Conversion/1 -> Reset_Logic/4(Extn_Reset)

== system motorcontrol_19a/Motor_Control4/Subsystem/Open Loop Start-Up/Subsystem1 ==
  m : Inport
  Theta : Inport  Port=2
  Constant : Constant  Value=0  OutDataTypeStr=Inherit: Inherit via back propagation  SampleTime=-1
  Data Type Duplicate : DataTypeDuplicate  NumInputPorts=3
  Sine-Cosine Lookup : Subsystem  mask{N_points=1024}
      mask prompts: N_points "Number of data points for lookup table:"
      mask init: same as motorcontrol_19a/Motor_Control4/Subsystem/Closed_Loop/Sine-Cosine Lookup
      mask DialogControl DescGroupVar Prompt: Sine-Cosine Lookup
      mask DialogControl DescTextVar Prompt: Implement sine and cosine functions using a lookup table approach for optimized performance on target hardware.
      mask Display: fprintf('Sin-Cos\n LUT');
  Subsystem1 : Subsystem  mask(Inverse Clarke Transform){}
      mask help:
      | <p>Compute Inverse Clarke transformation on balanced 2-phase orthogonal inputs into balanced 3-phase outputs.
      | <br><br>
      | The block accepts &alpha;-&beta; axis components and outputs corresponding 3-phase outputs, where phase-a axis is aligned with &alpha;-axis.</p>
      mask Display: fprintf('Inverse Clarke\n Transform');
  Subsystem2 : Subsystem  mask(Inverse Park Transform){AxisAlignment=D-axis}
      mask prompts: AxisAlignment "Alpha (phase-a ) axis alignment:"
      mask help:
      | <p>Compute Inverse Park transformation on rotating reference frame inputs into stationary reference frame outputs.
      | <br><br>
      | The block accepts the following:
      | <ul>
      | <li>d-q axis components in rotating reference frame</li>
      | <li>Sine and cosine values of corresponding angle of transformation</li>
      | </ul>
      | The block outputs &alpha;-&beta; axis components in stationary reference frame.
      | <br><br>
      | D-axis alignment with alpha (phase-a) is popular in motor control theory while Q-axis alignment with alpha (phase-a) is more suitable for power conversion applications.</p>
      mask init:
      | dlgSett.Offset = 0;
      | 
      | switch AxisAlignment
      |     case 'Q-axis'
      |         dlgSett.Offset = 90;
      |     case 'D-axis'
      |         dlgSett.Offset = 0;
      |     otherwise
      | end
      mask TypeOptions AxisAlignment: D-axis | Q-axis
      mask Display: fprintf('Inverse Park\n Transform');
  Unary Minus : UnaryMinus
  Va1 : Outport  VectorParamsAs1DForOutWhenUnconnected=off
  Vb1 : Outport  Port=2  VectorParamsAs1DForOutWhenUnconnected=off
  Vc1 : Outport  Port=3  VectorParamsAs1DForOutWhenUnconnected=off
  wires:
  Subsystem1/3(c) -> Vc1/1
  Subsystem2/1(Alpha) -> Subsystem1/1(In1)  "V_alpha"
  Theta/1 -> Sine-Cosine Lookup/1(Theta), Data Type Duplicate/2  "Eps"
  m/1 -> Unary Minus/1, Data Type Duplicate/1
  Unary Minus/1 -> Subsystem2/2(Qs)
  Subsystem2/2(Beta) -> Subsystem1/2(In2)  "V_beta"
  Subsystem1/1(a) -> Va1/1
  Subsystem1/2(b) -> Vb1/1
  Constant/1 -> Subsystem2/1(Ds), Data Type Duplicate/3
  Sine-Cosine Lookup/1(sin) -> Subsystem2/3(sin)
  Sine-Cosine Lookup/2(cos) -> Subsystem2/4(cos)

== system motorcontrol_19a/Motor_Control1/PMSM/Subsystem/Subsystem/Subsystem ==
  Abc : Inport
  Add : Sum  Inputs=+++
  Add1 : Sum
  Demux : Demux  Outputs=3
  Gain : Gain  Gain=2/3
  Gain1 : Gain  Gain=-1/3
  Gain2 : Gain  Gain=sqrt(3)/3
  Gain3 : Gain  Gain=-sqrt(3)/3
  Gain4 : Gain  Gain=-1/3
  Alpha : Outport  VectorParamsAs1DForOutWhenUnconnected=off
  Beta : Outport  Port=2  VectorParamsAs1DForOutWhenUnconnected=off
  wires:
  Gain4/1 -> Add/3
  Add/1 -> Alpha/1
  Demux/3 -> Gain3/1, Gain4/1
  Gain1/1 -> Add/2
  Gain2/1 -> Add1/1
  Demux/2 -> Gain2/1, Gain1/1
  Gain3/1 -> Add1/2
  Add1/1 -> Beta/1
  Abc/1 -> Demux/1
  Gain/1 -> Add/1
  Demux/1 -> Gain/1

== system motorcontrol_19a/Motor_Control1/PMSM/Subsystem/Subsystem/Subsystem1 ==
  Alpha : Inport
  Beta : Inport  Port=2
  SinTheta : Inport  Port=3
  CosTheta : Inport  Port=4
  Add : Sum  Inputs=-+
  Add1 : Sum
  Alpha1 : InportShadow
  Beta1 : InportShadow  Port=2
  CosTheta1 : InportShadow  Port=4
  Product{,1..3} (4 alike) : Product  RndMeth=Zero
  SineTheta1 : InportShadow  Port=3
  DSyn : Outport  VectorParamsAs1DForOutWhenUnconnected=off
  QSyn : Outport  Port=2  VectorParamsAs1DForOutWhenUnconnected=off
  wires:
  Product/1 -> Add/1
  Product1/1 -> Add/2
  Beta1/1 -> Product1/1
  Alpha1/1 -> Product/1
  Add/1 -> QSyn/1
  Beta/1 -> Product3/1
  Product2/1 -> Add1/1
  SinTheta/1 -> Product3/2
  Add1/1 -> DSyn/1
  Alpha/1 -> Product2/1
  CosTheta/1 -> Product2/2
  Product3/1 -> Add1/2
  CosTheta1/1 -> Product1/2
  SineTheta1/1 -> Product/2

== system motorcontrol_19a/Motor_Control1/PMSM/Subsystem/Subsystem/Subsystem2 ==
  VdSyn : Inport
  VqSyn : Inport  Port=2
  RotorElecSpd : Inport  Port=3
  Id cal : Subsystem
  Iq cal : Subsystem
  IdSyn : Outport  VectorParamsAs1DForOutWhenUnconnected=off
  IqSyn : Outport  Port=2  VectorParamsAs1DForOutWhenUnconnected=off
  wires:
  Iq cal/1(Iq) -> IqSyn/1, Id cal/1(Iq)
  Id cal/1(Id) -> IdSyn/1, Iq cal/1(Id)
  VdSyn/1 -> Id cal/3(Vd)
  VqSyn/1 -> Iq cal/2(Vq)
  RotorElecSpd/1 -> Id cal/2(we), Iq cal/3(we)

== system motorcontrol_19a/Motor_Control1/PMSM/Subsystem/Subsystem/Subsystem3 ==
  DSyn : Inport
  QSyn : Inport  Port=2
  SinTheta : Inport  Port=3
  CosTheta : Inport  Port=4
  Add : Sum
  Add1 : Sum  Inputs=+-
  CosTheta1 : InportShadow  Port=4
  DSyn1 : InportShadow
  Product{,1..3} (4 alike) : Product  RndMeth=Zero
  QSyn1 : InportShadow  Port=2
  SinTheta1 : InportShadow  Port=3
  Alpha : Outport  VectorParamsAs1DForOutWhenUnconnected=off
  Beta : Outport  Port=2  VectorParamsAs1DForOutWhenUnconnected=off
  wires:
  DSyn1/1 -> Product/1
  SinTheta1/1 -> Product/2
  Product2/1 -> Add1/1
  QSyn1/1 -> Product1/1
  Product1/1 -> Add/2
  Product/1 -> Add/1
  Add1/1 -> Alpha/1
  CosTheta1/1 -> Product1/2
  CosTheta/1 -> Product2/2
  QSyn/1 -> Product3/1
  DSyn/1 -> Product2/1
  Add/1 -> Beta/1
  SinTheta/1 -> Product3/2
  Product3/1 -> Add1/2

== system motorcontrol_19a/Motor_Control1/PMSM/Subsystem/Subsystem/Subsystem4 ==
  Alpha : Inport
  Beta : Inport  Port=2
  Gain1 : Gain  Gain=-1/2
  Gain2 : Gain  Gain=-1/2
  Gain3 : Gain  Gain=sqrt(3)/2
  Gain4 : Gain  Gain=-sqrt(3)/2
  Subtract1 : Sum
  Subtract2 : Sum
  A : Outport  VectorParamsAs1DForOutWhenUnconnected=off
  B : Outport  Port=2  VectorParamsAs1DForOutWhenUnconnected=off
  C : Outport  Port=3  VectorParamsAs1DForOutWhenUnconnected=off
  wires:
  Gain4/1 -> Subtract2/2
  Beta/1 -> Gain4/1, Gain3/1
  Alpha/1 -> A/1, Gain2/1, Gain1/1
  Subtract2/1 -> C/1
  Gain1/1 -> Subtract2/1
  Gain2/1 -> Subtract1/1
  Subtract1/1 -> B/1
  Gain3/1 -> Subtract1/2

== system motorcontrol_19a/Motor_Control1/PMSM/Subsystem/Subsystem/Subsystem5 ==
  Iq : Inport
  Id : Inport  Port=2
  1.5 P : Gain  Gain=1.5*P  OutDataTypeStr=dataType  RndMeth=Simplest
  Add : Sum
  Add1 : Sum  Inputs=+-
  Constant : Constant  Value=Ld
  Constant1 : Constant  Value=Lq
  Gain1 : Gain  Gain=FluxPM
  Product : Product
  Product1 : Product
  Te : Outport
  wires:
  1.5 P/1 -> Te/1  "Te"
  Iq/1 -> Product/1, Gain1/1  "Iq"
  Id/1 -> Product/2  "Id"
  Add/1 -> 1.5 P/1
  Gain1/1 -> Add/1
  Constant/1 -> Add1/1
  Constant1/1 -> Add1/2
  Product/1 -> Product1/1
  Add1/1 -> Product1/2
  Product1/1 -> Add/2

== system motorcontrol_19a/Motor_Control1/PMSM/Subsystem/Subsystem1/Subsystem ==
  In1 : Inport
  Add : Sum
  Add1 : Sum
  Compare To Constant : simulink/Logic and Bit Operations/Compare To Constant  relop=<=  const=U  OutDataTypeStr=boolean
  Compare To Constant1 : simulink/Logic and Bit Operations/Compare To Constant  relop=>=  const=L  OutDataTypeStr=boolean
  Constant1 : Constant  Value=U-L  OutDataTypeStr=single  SampleTime=-1
  Constant3 : Constant  Value=U-L  OutDataTypeStr=single  SampleTime=-1
  Gain1 : Gain  Gain=Ts
  Subtract : Sum  Inputs=+-
  Switch : Switch  Criteria=u2 > Threshold  OutDataTypeStr=single
  Switch1 : Switch  Criteria=u2 > Threshold  OutDataTypeStr=single
  Unit Delay : UnitDelay  InitialCondition=Ic  SampleTime=-1  HasFrameUpgradeWarning=on
  Out1 : Outport  VectorParamsAs1DForOutWhenUnconnected=off
  wires:
  Switch1/1 -> Add/2, Out1/1
  Unit Delay/1 -> Switch/1, Subtract/1, Compare To Constant1/1, Add1/1, Compare To Constant/1
  Subtract/1 -> Switch/3
  Switch/1 -> Switch1/1
  Compare To Constant/1 -> Switch/2
  Compare To Constant1/1 -> Switch1/2
  Constant1/1 -> Add1/2
  Constant3/1 -> Subtract/2
  In1/1 -> Gain1/1
  Add1/1 -> Switch1/3
  Add/1 -> Unit Delay/1
  Gain1/1 -> Add/1

== system motorcontrol_19a/Motor_Control1/PMSM/Subsystem/Subsystem2/Subsystem ==
  PwrTrnsfrd : Inport
  PwrNotTrnsfrd : Inport  Port=2
  PwrStored : Inport  Port=3
  Bus Creator : BusCreator  Inputs=3
  Signal Specification : SignalSpecification  Unit=W
  PwrInfo : Outport  VectorParamsAs1DForOutWhenUnconnected=off
  wires:
  Signal Specification/1 -> PwrInfo/1  "PwrInfo"
  PwrStored/1 -> Bus Creator/3  "PwrStored"
  Bus Creator/1 -> Signal Specification/1
  PwrNotTrnsfrd/1 -> Bus Creator/2  "PwrNotTrnsfrd"
  PwrTrnsfrd/1 -> Bus Creator/1  "PwrTrnsfrd"

== system motorcontrol_19a/Motor_Control4/Input Scaling/ Calculate Position and Speed/Subsystem2/PositionNoReset ==
  Index : Inport
  Count : Inport  Port=2
  Action Port : ActionPort
  CountsPerRevolution : Constant  Value=EncoderSlitsPerRevolution*4  OutDataTypeStr=Inherit: Inherit via back propagation
  MinMax : MinMax  Inputs=2  RndMeth=Simplest  ZeroCross=off
  Sum3 : Sum  Inputs=+-|  OutDataTypeStr=Inherit: Same as accumulator  RndMeth=Simplest
  Sum7 : Sum  Inputs=|++  OutDataTypeStr=Inherit: Same as accumulator  RndMeth=Simplest
  Position : Outport  VectorParamsAs1DForOutWhenUnconnected=off
  wires:
  Sum3/1 -> MinMax/1, Sum7/1
  Count/1 -> Sum3/1
  Index/1 -> Sum3/2
  CountsPerRevolution/1 -> Sum7/2
  Sum7/1 -> MinMax/2
  MinMax/1 -> Position/1

== system motorcontrol_19a/Motor_Control4/Input Scaling/ Calculate Position and Speed/Subsystem2/PositionResetatIndex ==
  Count : Inport
  Action Port : ActionPort
  Position : Outport  VectorParamsAs1DForOutWhenUnconnected=off
  wires:
  Count/1 -> Position/1

== system motorcontrol_19a/Motor_Control4/Input Scaling/ Calculate Position and Speed/Subsystem3/Subsystem ==
  ϴm : Inport
  In2 : Inport  Port=2
  If : If  NumInputs=2  IfExpression=u1 <= u2
  Merge : Merge
  Subsystem : Subsystem
  Subsystem1 : Subsystem
  Out1 : Outport
  wires:
  Merge/1 -> Out1/1
  If/2 -> Subsystem1/Action
  Subsystem/1(Out1) -> Merge/1
  ϴm/1 -> If/1, Subsystem/1(ϴm), Subsystem1/1(ϴm)
  If/1 -> Subsystem/Action
  Subsystem1/1(Out1) -> Merge/2
  In2/1 -> Subsystem/2(In2), Subsystem1/2(In2), If/2

== system motorcontrol_19a/Motor_Control4/Input Scaling/ Calculate Position and Speed/Subsystem3/Subsystem1 ==
  In1 : Inport
  Add : Sum  Inputs=-+  OutDataTypeStr=Inherit: Inherit via back propagation  RndMeth=Simplest
  Floor : Rounding
  Multiply : Gain  Gain=1/maxAngleIn  RndMeth=Simplest  OutDataTypeStr=Inherit: Same as input
  Multiply1 : Gain  Gain=maxAngleIn  OutDataTypeStr=Inherit: Inherit via back propagation  RndMeth=Simplest
  Number of pole pairs : Gain  Gain=NrPP  RndMeth=Simplest  OutDataTypeStr=Inherit: Same as input
  Out1 : Outport
  ϴe : Outport  Port=2
  wires:
  Multiply1/1 -> Add/1
  Number of pole pairs/1 -> Multiply/1, Add/2
  Add/1 -> ϴe/1, Out1/1
  Floor/1 -> Multiply1/1
  Multiply/1 -> Floor/1
  In1/1 -> Number of pole pairs/1

== system motorcontrol_19a/Motor_Control4/Subsystem/Closed_Loop/Current_Controllers1/FeedForward Decoupling Compensation ==
  d_current measured : Inport
  Electrical_speed measured : Inport  Port=2
  q_current measured : Inport  Port=3
  Add : Sum
  Constant : Constant  Value=pmsm.Ld  OutDataTypeStr=Inherit: Inherit via back propagation  SampleTime=-1
  Constant1 : Constant  Value=pmsm.FluxPM  OutDataTypeStr=Inherit: Inherit via back propagation  SampleTime=-1
  Constant2 : Constant  Value=pmsm.Lq  OutDataTypeStr=Inherit: Inherit via back propagation  SampleTime=-1
  Data Type Duplicate : DataTypeDuplicate  NumInputPorts=6
  Product4 : Product  Inputs=3
  Product5 : Product
  Product6 : Product
  Unary Minus : UnaryMinus
  q_voltage_compensation : Outport
  d_voltage_compensation : Outport  Port=2
  wires:
  Add/1 -> Product6/2
  Electrical_speed measured/1 -> Product4/3, Product6/1, Data Type Duplicate/2
  Product5/1 -> Add/1
  d_current measured/1 -> Product5/1, Data Type Duplicate/3
  Constant2/1 -> Product4/1, Data Type Duplicate/6
  Constant/1 -> Data Type Duplicate/4, Product5/2
  Constant1/1 -> Data Type Duplicate/5, Add/2
  q_current measured/1 -> Product4/2, Data Type Duplicate/1
  Product4/1 -> Unary Minus/1
  Unary Minus/1 -> q_voltage_compensation/1
  Product6/1 -> d_voltage_compensation/1

== system motorcontrol_19a/Motor_Control4/Subsystem/Closed_Loop/Current_Controllers1/Subsystem ==
  Vd_ref : Inport
  Vq_ref : Inport  Port=2
  Data Type Duplicate : DataTypeDuplicate
  Demux : Demux  Outputs=2
  Gain : Gain  Gain=Vmax  OutDataTypeStr=Inherit: Same as input
  Math Function2 : Math  Operator=reciprocal  RndMeth=Simplest
  Mux : Mux  Inputs=2
  Product : Product  RndMeth=Simplest  OutDataTypeStr=Inherit: Same as first input
  Product1 : Product  RndMeth=Simplest  OutDataTypeStr=Inherit: Same as first input
  Product2 : Product  OutDataTypeStr=Inherit: Same as first input
  Sqrt : Sqrt  IntermediateResultsDataTypeStr=Inherit: Inherit from input  SaturateOnIntegerOverflow=on
  Sum2 : Sum  OutDataTypeStr=Inherit: Same as first input
  Switch : Switch  Threshold=Vmax  ZeroCross=off
  Vd_sat : Outport  VectorParamsAs1DForOutWhenUnconnected=off
  Vq_sat : Outport  Port=2  VectorParamsAs1DForOutWhenUnconnected=off
  wires:
  Vd_ref/1 -> Mux/1, Product/2, Product/1, Data Type Duplicate/1
  Demux/1 -> Vd_sat/1
  Product1/1 -> Sum2/2
  Product/1 -> Sum2/1
  Sum2/1 -> Sqrt/1
  Gain/1 -> Product2/1
  Math Function2/1 -> Gain/1
  Vq_ref/1 -> Mux/2, Product1/2, Product1/1, Data Type Duplicate/2
  Mux/1 -> Switch/3, Product2/2
  Product2/1 -> Switch/1
  Demux/2 -> Vq_sat/1
  Sqrt/1 -> Switch/2, Math Function2/1
  Switch/1 -> Demux/1
